simulink model "ABLF_SOC_benchmark"  (R2021b)
settings: Solver=FixedStepAuto  StartTime=0.0  StopTime=100  FixedStep=0.0001  RelTol=1e-3
values from neighbouring files (symbols this model uses):
  a = 2    [ABLF_SLDO_benchmark_Start.m]    (also in ABLF_SOC_benchmark_Start.m)
  amp = pi/2    (= 1.57079632679)    [ABLF_SLDO_benchmark_Start.m]    (also in ABLF_SOC_benchmark_Start.m)
  f1 = 0    [ABLF_SLDO_benchmark_Start.m]    (also in ABLF_SOC_benchmark_Start.m)
  g1 = 1    [ABLF_SLDO_benchmark_Start.m]    (also in ABLF_SOC_benchmark_Start.m)
  g2 = Kt/J    (= 0.530555555556)    [ABLF_SLDO_benchmark_Start.m]    (also in ABLF_SOC_benchmark_Start.m)
  g3 = 1/L    (= 333.333333333)    [ABLF_SLDO_benchmark_Start.m]    (also in ABLF_SOC_benchmark_Start.m)
  J = 1.8*10^(-2)    (= 0.018)    [ABLF_SLDO_benchmark_Start.m]    (also in ABLF_SOC_benchmark_Start.m)
  k = 2    [ABLF_SLDO_benchmark_Start.m]    (also in ABLF_SOC_benchmark_Start.m)
  k1 = 6.2718    [ABLF_SLDO_benchmark_Start.m]    (also in ABLF_SOC_benchmark_Start.m = 10)
  k2 = 2.3993e+03    (= 2399.3)    [ABLF_SLDO_benchmark_Start.m]    (also in ABLF_SOC_benchmark_Start.m = 1)
  k3 = 31.9167    [ABLF_SLDO_benchmark_Start.m]    (also in ABLF_SOC_benchmark_Start.m = 10)
  ka1 = kcl1 - (-amp)    (= -0.429203673205)    [ABLF_SLDO_benchmark_Start.m]    (also in ABLF_SOC_benchmark_Start.m = kcl1 - (-amp))
  kb1 = kcl2 - (amp)    (= 0.429203673205)    [ABLF_SLDO_benchmark_Start.m]    (also in ABLF_SOC_benchmark_Start.m = kcl2 - (amp))
  Ke = 9.55*10^(-3)    (= 0.00955)    [ABLF_SLDO_benchmark_Start.m]    (also in ABLF_SOC_benchmark_Start.m)
  Kt = 9.55*10^(-3)    (= 0.00955)    [ABLF_SLDO_benchmark_Start.m]    (also in ABLF_SOC_benchmark_Start.m)
  L = 0.003    [ABLF_SLDO_benchmark_Start.m]    (also in ABLF_SOC_benchmark_Start.m = 1)
  maxKd = 100    [ABLF_SOC_benchmark_Start.m]
  maxKi = 1    [ABLF_SOC_benchmark_Start.m]
  maxKp = 100    [ABLF_SOC_benchmark_Start.m]
  minKd = 0.001    [ABLF_SOC_benchmark_Start.m]
  minKi = 0.01    [ABLF_SOC_benchmark_Start.m]
  minKp = 0.01    [ABLF_SOC_benchmark_Start.m]
  mu1 = 1.8    [ABLF_SLDO_benchmark_Start.m]    (also in ABLF_SOC_benchmark_Start.m)
  optimPeriod = 0.5    [ABLF_SOC_benchmark_Start.m]
  OVLim = 0.15    [ABLF_SOC_benchmark_Start.m]
  R = 0.21    [ABLF_SLDO_benchmark_Start.m]    (also in ABLF_SOC_benchmark_Start.m)
  refSignalPeriod = 0.5    [ABLF_SOC_benchmark_Start.m]
  resetThreshold = 0.1    [ABLF_SOC_benchmark_Start.m]
  t2 = 0.012    [ABLF_SLDO_benchmark_Start.m]    (also in ABLF_SOC_benchmark_Start.m = 0.0005)
  t3 = 0.012    [ABLF_SLDO_benchmark_Start.m]    (also in ABLF_SOC_benchmark_Start.m = 0.01)
  TSLim = 0.1    [ABLF_SOC_benchmark_Start.m]
  W1 = 0.1    [ABLF_SOC_benchmark_Start.m]
  W2 = 1    [ABLF_SOC_benchmark_Start.m]
  W3 = 0.109    [ABLF_SOC_benchmark_Start.m]
undefined symbols (not defined in the file or in its folder): DiscIntNeverNeededParam
libraries: dspmathops x2
settings Model: Creator=mcald  LastModifiedBy=mcald
settings DataIOCC: ReturnWorkspaceOutputs=off

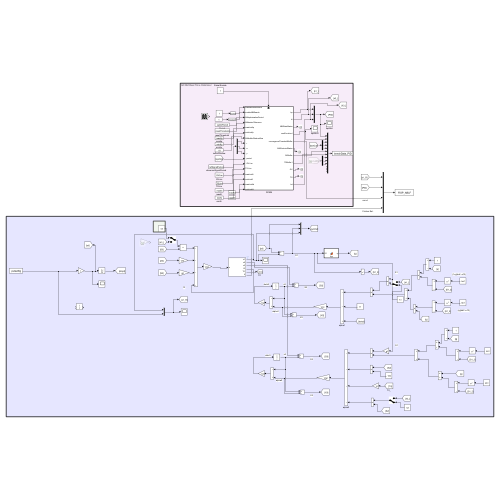
[thumbnail: Simulink's stored preview of the top-level diagram]
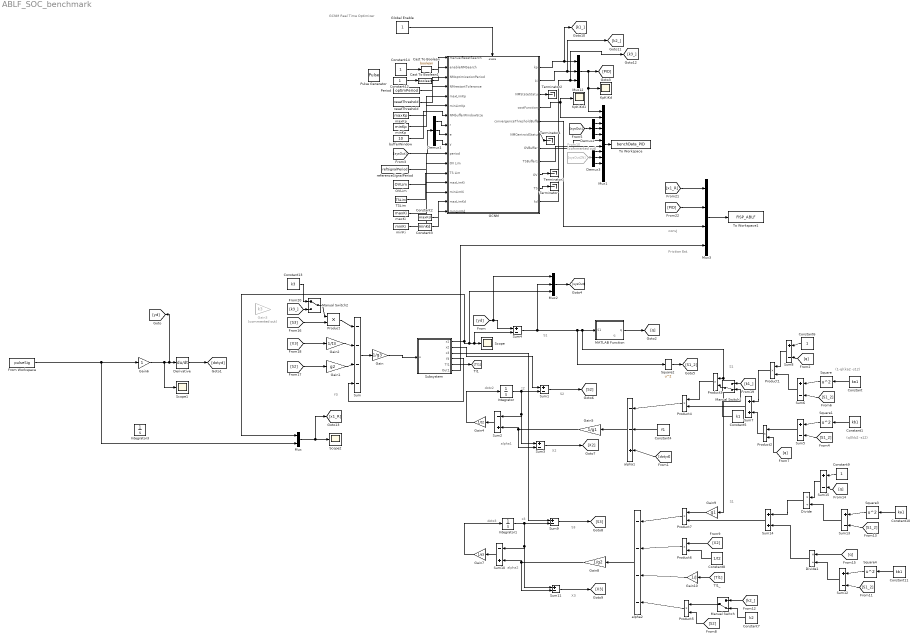
== system ABLF_SOC_benchmark ==
  note: Friction Est.
  note: convJ
  note: GCNM Real Time Optimizer
  note: S1
  note: alpha2
  note: S2
  note: z3
  note: f3
  note: dotz3
  note: (q)(kb2 -s12)
  note: X3
  note: S3
  note: S1
  note: S1
  note: q
  note: z2
  note: X2
  note: dotz2
  note: alpha1
  note: (1-q)(ka2 -s12)
  Cast To Boolean : DataTypeConversion  OutDataTypeStr=boolean
  Cast To Boolean1 : DataTypeConversion  OutDataTypeStr=boolean
  Constant : Constant  Value=ka1
  Constant1 : Constant  Value=kb1
  Constant10 : Constant  Value=ka1
  Constant11 : Constant  Value=kb1
  Constant12 : Constant  OutDataTypeStr=boolean
  Constant13 : Constant  Value=k3
  Constant14 : Constant
  Constant2 : Constant  Value=maxKd
  Constant3 : Constant  Value=minKd
  Constant4 : Constant  Value=f1
  Constant5 : Constant  Value=k1
  Constant6 : Constant
  Constant7 : Constant  Value=k2
  Constant8 : Constant  Value=1/t2
  Constant9 : Constant
  Demux1 : Demux  Outputs=3
  Demux2 : Demux  Outputs=3
  Demux3 : Demux  Outputs=3
  Derivative : Derivative
  Divide : Product  Inputs=*/
  Divide1 : Product  Inputs=*/
  From Workspace : FromWorkspace  VariableName=pulseSig
  From10 : From  Commented=on  GotoTag=sysOutZN
  GCNM : Subsystem
  Gain : Gain  Gain=1/g3
  Gain1 : Gain  Gain=g2
  Gain10 : Gain  Gain=1/J
  Gain2 : Gain  Gain=1/t3
  Gain3 : Gain  Commented=on  Gain=k3
  Gain4 : Gain  Gain=1/t2
  Gain5 : Gain  Gain=1/g1
  Gain6 : Gain
  Gain7 : Gain  Gain=1/t3
  Gain8 : Gain  Gain=1/g2
  Gain9 : Gain  Gain=g1
  Global Enable : Constant
  Integrator : Integrator  InitialCondition=-5.0078
  Integrator1 : Integrator  InitialCondition=-2094.2231
  Integrator3 : Integrator  InitialCondition=0.1
  KpKiKd : Scope
  KpKiKd1 : Scope
  MATLAB Function : MATLAB Function  TreatAsAtomicUnit=on
  Manual Switch : ManualSwitch  CurrentSetting=0
  Manual Switch1 : ManualSwitch  CurrentSetting=0
  Manual Switch2 : ManualSwitch
  Mux : Mux  Inputs=2
  Mux1 : Mux  Inputs=12
  Mux12 : Mux  Inputs=3
  Mux2 : Mux  Inputs=3
  Mux3 : Mux
  OVLim : Constant  Value=OVLim
  Period : Constant  Value=optimPeriod  OutDataTypeStr=double
  Product{,1..7} (8 alike) : Product
  Pulse Generator : DiscretePulseGenerator  PulseType=Time based  Period=20  PulseWidth=0.1
  Scope : Scope
  Scope1 : Scope
  Scope2 : Scope
  Square{,1..4} (5 alike) : Math  Operator=square  SaturateOnIntegerOverflow=on
  Subsystem : Subsystem
  Sum : Sum  Inputs=-|-|-|-
  Sum{1,3..6,8..9,11..13,15} (11 alike) : Sum  Inputs=+|-
  Sum10 : Sum  Inputs=-|+
  Sum14 : Sum  Inputs=+|+
  Sum2 : Sum  Inputs=-|+
  Sum7 : Sum  Inputs=+|+
  TSLim : Constant  Value=TSLim
  Terminator{,1..2,4} (4 alike) : Terminator
  To Workspace : ToWorkspace  VariableName=benchData_PID  SaveFormat=Timeseries  SampleTime=-1
  To Workspace1 : ToWorkspace  VariableName=FISP_ABLF  SaveFormat=Timeseries  SampleTime=-1
  alpha1 : Sum  Inputs=-|-|+
  alpha2 : Sum  Inputs=-|-|-|-
  bufferWindow : Constant  Value=10  OutDataTypeStr=uint16
  maxKi : Constant  Value=maxKi  VectorParams1D=off  OutDataTypeStr=double
  maxKp : Constant  Value=maxKp  OutDataTypeStr=double
  minKi : Constant  Value=minKi  OutDataTypeStr=double
  minKp : Constant  Value=minKp  OutDataTypeStr=double
  referenceSignalPeriod : Constant  Value=refSignalPeriod
  resetThreshold : Constant  Value=resetThreshold
  wires:
  GCNM/9(OV) -> Terminator1/1
  Constant2/1 -> GCNM/16(maxLimKd)
  maxKp/1 -> GCNM/5(maxLimKp)
  Demux3/3 -> Mux1/10
  GCNM/3(NMStateStatus) -> Terminator2/1
  minKp/1 -> GCNM/6(minLimKp)
  Constant3/1 -> GCNM/17(minLimKd)
  [sysOut] -> Demux1/1
  bufferWindow/1 -> GCNM/7(NMbufferWindowSize)
  GCNM/6(NMCentroidStatus) -> Terminator4/1
  Cast To Boolean1/1 -> GCNM/2(enableNMSearch)
  Mux1/1 -> To Workspace/1
  OVLim/1 -> GCNM/12("  OV Lim")
  Demux3/2 -> Mux1/9
  Constant12/1 -> Cast To Boolean1/1
  From10/1 -> Demux3/1
  GCNM/4(costFunctionJ) -> Mux1/2, KpKiKd1/1
  Demux3/1 -> Mux1/8
  GCNM/7(OVBuffer) -> Mux1/6
  GCNM/8(TSBuffer1) -> Mux1/7
  GCNM/11(kd) -> [k3_], Mux12/3
  Demux2/3 -> Mux1/5
  TSLim/1 -> GCNM/13(TS Lim)
  GCNM/1("  kp") -> [k1_], Mux12/1
  referenceSignalPeriod/1 -> GCNM/11("  period")
  Mux12/1 -> Mux1/1, KpKiKd/1, [PID]
  Demux1/3 -> GCNM/10("  y")
  GCNM/10(TS) -> Terminator/1
  Cast To Boolean/1 -> GCNM/1(manualResetSearch)
  Demux2/1 -> Mux1/3
  Demux1/1 -> GCNM/8("  r")
  resetThreshold/1 -> GCNM/4(NMrestartTolerance)
  Demux2/2 -> Mux1/4
  maxKi/1 -> GCNM/14(maxLimKi)
  Global Enable/1 -> GCNM/Enable
  Demux1/2 -> GCNM/9("  e")
  Period/1 -> GCNM/3(NMoptimizationPeriod)
  GCNM/2("  ki") -> [k2_], Mux12/2
  minKi/1 -> GCNM/15(minLimKi)
  Constant14/1 -> Cast To Boolean/1
  [sysOut] -> Demux2/1
  [q] -> Sum8/2
  Sum7/1 -> Product4/2
  Constant1/1 -> Square1/1
  MATLAB Function/1(q) -> [q]
  [S1_2] -> Sum12/2
  Subsystem/4(f3) -> Sum/4
  Gain5/1 -> Sum2/2, Sum3/2
  [Tl1] -> Gain10/1
  Constant/1 -> Square/1
  [S2] -> Gain1/1
  Divide/1 -> Sum14/1
  Square3/1 -> Sum13/1
  Square2/1 -> [S1_2]
  [q] -> Divide1/1
  [X3] -> Gain2/1
  Constant11/1 -> Square4/1
  Subsystem/3(x3) -> Sum9/1
  Mux/1 -> [x1_R], Scope2/1
  Sum1/1 -> [S2]
  [q] -> Sum15/2
  Gain9/1 -> Product7/1
  [X2] -> Product6/1
  Sum11/1 -> [X3]
  Constant8/1 -> Product6/2
  Subsystem/2(x2) -> Sum1/1
  [yd] -> Mux2/1, Sum4/1
  Sum15/1 -> Divide/1
  [S1_2] -> Sum13/2
  Constant9/1 -> Sum15/1
  Constant6/1 -> Sum8/1
  Divide1/1 -> Sum14/2
  Product7/1 -> alpha2/1
  Product5/1 -> alpha2/4
  [S2] -> Product5/2
  Gain8/1 -> Sum10/2, Sum11/2
  Square1/1 -> Sum5/1
  Gain7/1 -> Integrator1/1
  Integrator1/1 -> Sum11/1, Sum10/1, Sum9/2
  Product2/1 -> Sum7/2
  Product1/1 -> Sum7/1
  Product6/1 -> alpha2/2
  alpha1/1 -> Gain5/1
  alpha2/1 -> Gain8/1
  Sum10/1 -> Gain7/1
  Sum5/1 -> Product2/1
  Integrator/1 -> Sum3/1, Sum2/1, Sum1/2
  Sum9/1 -> [S3]
  Subsystem/5(Tl1) -> [Tl1]
  [S1_2] -> Sum6/2
  [q] -> Product2/2
  Product4/1 -> alpha1/1
  Sum4/1 -> Square2/1, Gain9/1, Product3/1, MATLAB Function/1(S1), Mux2/2
  Sum3/1 -> [X2]
  Gain2/1 -> Sum/2
  Gain6/1 -> Derivative/1, [yd], Scope1/1
  Derivative/1 -> [dotyd]
  [S1_2] -> Sum5/2
  Square4/1 -> Sum12/1
  Constant4/1 -> alpha1/2
  Gain/1 -> Subsystem/1(u)
  Sum6/1 -> Product1/2
  Sum8/1 -> Product1/1
  Sum12/1 -> Divide1/2
  From Workspace/1 -> Mux/2, Gain6/1
  Gain1/1 -> Sum/3
  Gain4/1 -> Integrator/1
  Product/1 -> Sum/1
  Sum/1 -> Gain/1
  Mux2/1 -> [sysOut]
  Sum2/1 -> Gain4/1
  [dotyd] -> alpha1/3
  Square/1 -> Sum6/1
  Sum13/1 -> Divide/2
  Sum14/1 -> Product7/2
  Product3/1 -> Product4/1
  [S3] -> Product/2
  Constant10/1 -> Square3/1
  Gain10/1 -> alpha2/3
  Subsystem/1(x1) -> Mux2/3, Sum4/2, Scope/1, Mux/1
  Mux3/1 -> To Workspace1/1
  [x1_R] -> Mux3/1
  [PID] -> Mux3/2
  GCNM/5(convergenceThresholdBuffer) -> Mux3/3
  Subsystem/6(Out1) -> Mux3/4
  Manual Switch/1 -> Product5/1
  [k2_] -> Manual Switch/1
  Constant7/1 -> Manual Switch/2
  Manual Switch1/1 -> Product3/2
  [k1_] -> Manual Switch1/1
  Constant5/1 -> Manual Switch1/2
  [k3_] -> Manual Switch2/2
  Constant13/1 -> Manual Switch2/1
  Manual Switch2/1 -> Product/1

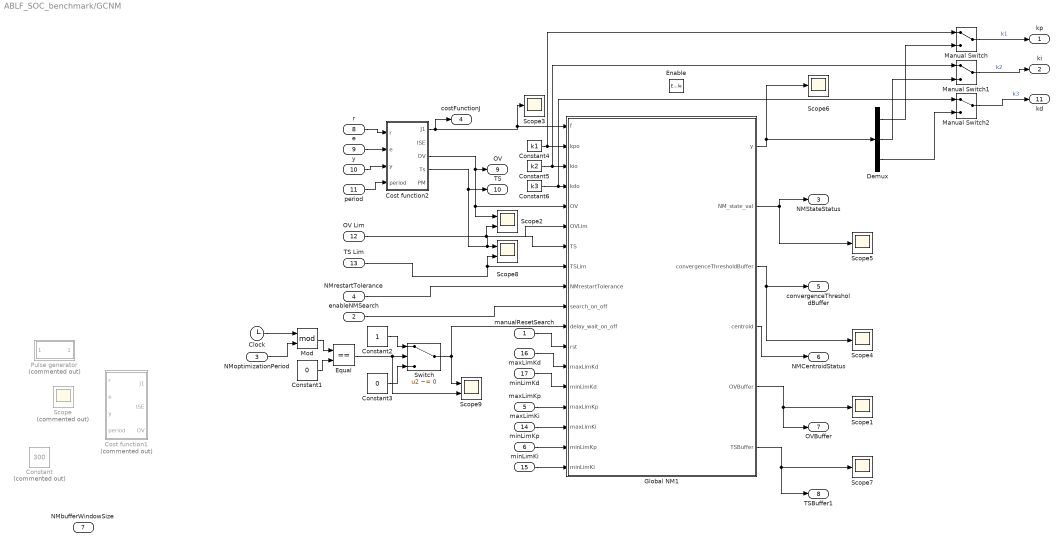
== system ABLF_SOC_benchmark/GCNM ==
  manualResetSearch : Inport  OutDataTypeStr=boolean
  enableNMSearch : Inport  Port=2  OutDataTypeStr=boolean
  NMoptimizationPeriod : Inport  Port=3  OutDataTypeStr=double
  NMrestartTolerance : Inport  Port=4
  maxLimKp : Inport  Port=5  OutDataTypeStr=double
  minLimKp : Inport  Port=6  OutDataTypeStr=double
  NMbufferWindowSize : Inport  Port=7  OutDataTypeStr=uint16
  "  r" : Inport  Port=8  OutDataTypeStr=double
  "  e" : Inport  Port=9  OutDataTypeStr=double
  "  y" : Inport  Port=10  OutDataTypeStr=double
  "  period" : Inport  Port=11  OutDataTypeStr=double
  "  OV Lim" : Inport  Port=12  OutDataTypeStr=double
  TS Lim : Inport  Port=13  OutDataTypeStr=double
  maxLimKi : Inport  Port=14  OutDataTypeStr=double
  minLimKi : Inport  Port=15  OutDataTypeStr=double
  maxLimKd : Inport  Port=16
  minLimKd : Inport  Port=17
  Enable : EnablePort
  Clock : Clock
  Constant : Constant  Commented=on  Value=300
  Constant1 : Constant  Value=0
  Constant2 : Constant
  Constant3 : Constant  Value=0
  Constant4 : Constant  Value=k1
  Constant5 : Constant  Value=k2
  Constant6 : Constant  Value=k3
  Cost function1 : Subsystem  Commented=on
  Cost function2 : Subsystem
  Demux : Demux  Outputs=3
  Equal : RelationalOperator  Operator===  RndMeth=Simplest
  Global NM1 : MATLAB Function  TreatAsAtomicUnit=on
  Manual Switch : ManualSwitch
  Manual Switch1 : ManualSwitch
  Manual Switch2 : ManualSwitch
  Mod : Math  Operator=mod  SaturateOnIntegerOverflow=on
  Pulse generator : Subsystem  Commented=on
  Scope : Scope  Commented=on
  Scope{1,3..7} (6 alike) : Scope
  Scope2 : Scope  NumInputPorts=2
  Scope8 : Scope  NumInputPorts=2
  Scope9 : Scope  NumInputPorts=2
  Switch : Switch  Criteria=u2 ~= 0
  "  kp" : Outport  OutDataTypeStr=double
  "  ki" : Outport  Port=2  OutDataTypeStr=double
  NMStateStatus : Outport  Port=3  OutDataTypeStr=double
  costFunctionJ : Outport  Port=4  OutDataTypeStr=double
  convergenceThresholdBuffer : Outport  Port=5  OutDataTypeStr=double
  NMCentroidStatus : Outport  Port=6  OutDataTypeStr=double
  OVBuffer : Outport  Port=7  OutDataTypeStr=double
  TSBuffer1 : Outport  Port=8  OutDataTypeStr=double
  OV : Outport  Port=9  OutDataTypeStr=double
  TS : Outport  Port=10  OutDataTypeStr=double
  kd : Outport  Port=11
  wires:
  NMrestartTolerance/1 -> Global NM1/9(NMrestartTolerance)
  manualResetSearch/1 -> Global NM1/12(rst)
  enableNMSearch/1 -> Global NM1/10(search_on_off)
  minLimKp/1 -> Global NM1/17(minLimKp)
  maxLimKp/1 -> Global NM1/15(maxLimKp)
  Global NM1/2(NM_state_val) -> NMStateStatus/1, Scope5/1
  Global NM1/3(convergenceThresholdBuffer) -> convergenceThresholdBuffer/1, Scope4/1
  Global NM1/4(centroid) -> NMCentroidStatus/1
  Global NM1/1(y) -> Scope6/1, Demux/1
  Constant5/1 -> Manual Switch1/1, Global NM1/3(kio)
  Cost function2/3(OV) -> OV/1, Scope2/1, Global NM1/5(OV)
  "  y"/1 -> Cost function2/3(y)
  "  e"/1 -> Cost function2/2(e)
  "  r"/1 -> Cost function2/1(r)
  Global NM1/5(OVBuffer) -> OVBuffer/1, Scope1/1
  "  period"/1 -> Cost function2/4(period)
  "  OV Lim"/1 -> Scope2/2, Global NM1/6(OVLim)
  Cost function2/4(Ts) -> TS/1, Global NM1/7(TS), Scope8/1
  TS Lim/1 -> Scope8/2, Global NM1/8(TSLim)
  Global NM1/6(TSBuffer) -> TSBuffer1/1, Scope7/1
  Cost function2/1(J1) -> Scope3/1, Global NM1/1(f), costFunctionJ/1
  Clock/1 -> Mod/1
  NMoptimizationPeriod/1 -> Mod/2
  Constant1/1 -> Equal/2
  Mod/1 -> Equal/1
  Constant2/1 -> Switch/1
  Constant3/1 -> Switch/3
  Switch/1 -> Scope9/1, Global NM1/11(delay_wait_on_off)
  Equal/1 -> Scope9/2, Switch/2
  maxLimKi/1 -> Global NM1/16(maxLimKi)
  minLimKi/1 -> Global NM1/18(minLimKi)
  maxLimKd/1 -> Global NM1/13(maxLimKd)
  minLimKd/1 -> Global NM1/14(minLimKd)
  Constant6/1 -> Manual Switch2/1, Global NM1/4(kdo)
  Constant4/1 -> Manual Switch/1, Global NM1/2(kpo)
  Manual Switch/1 -> "  kp"/1  "k1"
  Manual Switch2/1 -> kd/1  "k3"
  Manual Switch1/1 -> "  ki"/1  "k2"
  Demux/1 -> Manual Switch/2
  Demux/2 -> Manual Switch1/2
  Demux/3 -> Manual Switch2/2

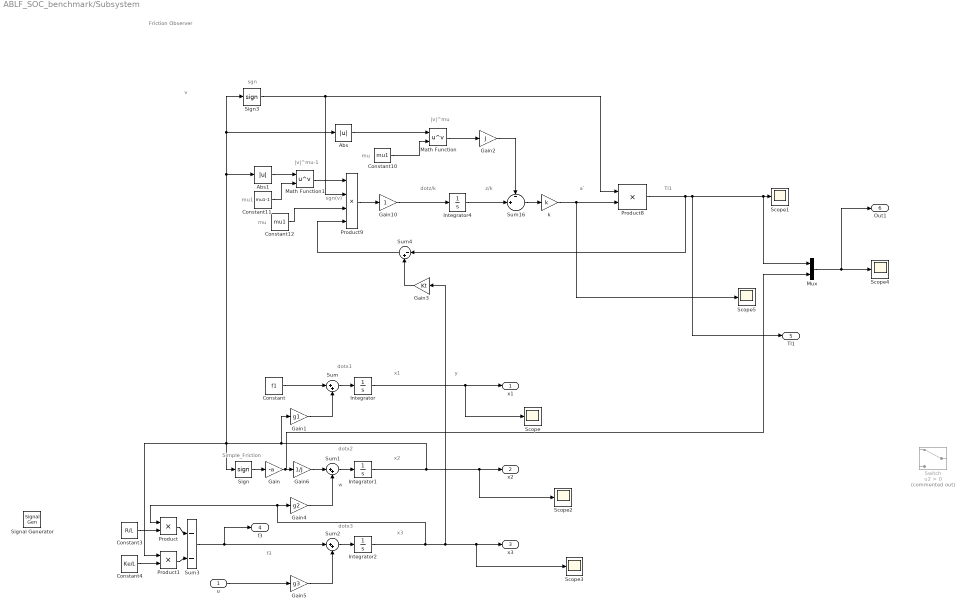
== system ABLF_SOC_benchmark/Subsystem ==
  note: Simple_Friction
  note: w
  note: f3
  note: y
  note: x1
  note: dotx1
  note: dotx2
  note: x2
  note: dotx3
  note: x3
  note: mu1
  note: dotz/k
  note: v
  note: mu
  note: a`
  note: z/k
  note: sgn
  note: Friction Observer
  note: mu
  note: |v|^mu-1
  note: sgn(v)
  note: |v|^mu
  note: Tl1
  u : Inport
  Abs : Abs
  Abs1 : Abs
  Constant : Constant  Value=f1
  Constant10 : Constant  Value=mu1
  Constant11 : Constant  Value=mu1-1
  Constant12 : Constant  Value=mu1
  Constant3 : Constant  Value=R/L
  Constant4 : Constant  Value=Ke/L
  Gain : Gain  Gain=-a
  Gain1 : Gain  Gain=g1
  Gain10 : Gain
  Gain2 : Gain  Gain=J
  Gain3 : Gain  Gain=Kt
  Gain4 : Gain  Gain=g2
  Gain5 : Gain  Gain=g3
  Gain6 : Gain  Gain=1/J
  Integrator : Integrator  InitialCondition=0.1
  Integrator1 : Integrator  InitialCondition=0.1
  Integrator2 : Integrator  InitialCondition=0.1
  Integrator4 : Integrator  InitialCondition=1
  Math Function : Math  Operator=pow  SaturateOnIntegerOverflow=on
  Math Function1 : Math  Operator=pow  SaturateOnIntegerOverflow=on
  Mux : Mux  Inputs=2
  Product : Product
  Product1 : Product
  Product8 : Product
  Product9 : Product  Inputs=4
  Scope{,1..5} (6 alike) : Scope
  Sign : Signum
  Sign3 : Signum
  Signal Generator : SignalGenerator  WaveForm=square  Amplitude=pi/2  Frequency=0.1  Units=rad/sec
  Sum : Sum  Inputs=|++
  Sum1 : Sum  Inputs=|++
  Sum16 : Sum  Inputs=-|+||
  Sum2 : Sum  Inputs=|++
  Sum3 : Sum  Inputs=-|-
  Sum4 : Sum  Inputs=|-+
  Switch : Switch  Commented=on  Criteria=u2 > Threshold
  k : Gain  Gain=k
  x1 : Outport
  x2 : Outport  Port=2
  x3 : Outport  Port=3
  f3 : Outport  Port=4
  Tl1 : Outport  Port=5
  Out1 : Outport  Port=6
  wires:
  Gain1/1 -> Sum/2
  Gain5/1 -> Sum2/2
  Integrator/1 -> Scope/1, x1/1
  Sum2/1 -> Integrator2/1
  Sum3/1 -> f3/1, Sum2/1
  Constant/1 -> Sum/1
  Sum1/1 -> Integrator1/1
  Integrator2/1 -> Gain3/1, Scope3/1, x3/1, Product/1, Gain4/1
  Sum/1 -> Integrator/1
  Constant3/1 -> Product/2
  Product/1 -> Sum3/1
  Product1/1 -> Sum3/2
  Constant4/1 -> Product1/2
  Integrator4/1 -> Sum16/2
  Abs1/1 -> Math Function1/1
  Math Function1/1 -> Product9/1
  Abs/1 -> Math Function/1
  Product9/1 -> Gain10/1
  Sum16/1 -> k/1
  Gain10/1 -> Integrator4/1
  Sign3/1 -> Product9/2, Product8/1
  Constant12/1 -> Product9/3
  Constant10/1 -> Math Function/2
  k/1 -> Scope5/1, Product8/2
  Constant11/1 -> Math Function1/2
  Sign/1 -> Gain/1
  Gain4/1 -> Sum1/2
  u/1 -> Gain5/1
  Math Function/1 -> Gain2/1
  Gain2/1 -> Sum16/1
  Mux/1 -> Out1/1, Scope4/1
  Product8/1 -> Sum4/1, Tl1/1, Mux/1, Scope1/1
  Integrator1/1 -> Gain1/1, Abs1/1, Abs/1, Sign3/1, Sign/1, Product1/1, Scope2/1, x2/1
  Gain3/1 -> Sum4/2
  Sum4/1 -> Product9/4
  Gain6/1 -> Sum1/1
  Gain/1 -> Mux/2, Gain6/1

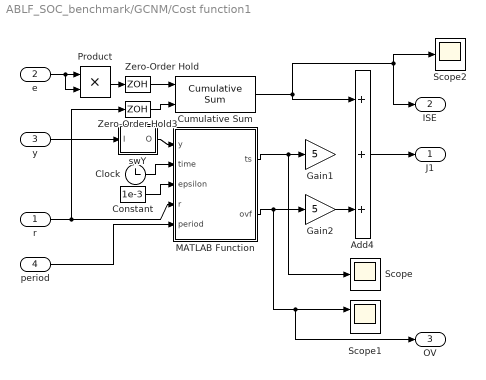
== system ABLF_SOC_benchmark/GCNM/Cost function1 ==
  r : Inport
  e : Inport  Port=2
  y : Inport  Port=3
  period : Inport  Port=4
  Add4 : Sum  Inputs=+++
  Clock : Clock
  Constant : Constant  Value=1e-3
  Cumulative Sum : dspmathops/Cumulative Sum  dim=Channels (running sum)  InputProcessing=Columns as channels (frame based)  reset_popup=Falling edge  roundingMode=Floor  overflowMode=off  outputDataTypeStr=Inherit: Same as accumulator  outputMin=[]  outputMax=[]  outputLastDataTypeStr=Inherit: Same as accumulator
  Gain1 : Gain  Gain=5
  Gain2 : Gain  Gain=5
  MATLAB Function : MATLAB Function  TreatAsAtomicUnit=on
  Product : Product
  Scope : Scope
  Scope1 : Scope  NumInputPorts=2
  Scope2 : Scope
  Zero-Order Hold : ZeroOrderHold  SampleTime=-1
  Zero-Order Hold3 : ZeroOrderHold  SampleTime=-1
  swY : Subsystem
  J1 : Outport
  ISE : Outport  Port=2
  OV : Outport  Port=3
  wires:
  period/1 -> MATLAB Function/5(period)
  Gain2/1 -> Add4/3
  Add4/1 -> J1/1
  y/1 -> swY/1(I)
  Constant/1 -> MATLAB Function/3(epsilon)
  Product/1 -> Zero-Order Hold/1
  Clock/1 -> MATLAB Function/2(time)
  swY/1(O) -> MATLAB Function/1(y)
  MATLAB Function/2(ovf) -> Gain2/1, Scope1/1, OV/1
  r/1 -> MATLAB Function/4(r), Zero-Order Hold3/1
  Zero-Order Hold/1 -> Cumulative Sum/1
  MATLAB Function/1(ts) -> Gain1/1, Scope/1
  e/1 -> Product/1, Product/2
  Zero-Order Hold3/1 -> Cumulative Sum/2
  Cumulative Sum/1 -> Scope2/1, ISE/1, Add4/1

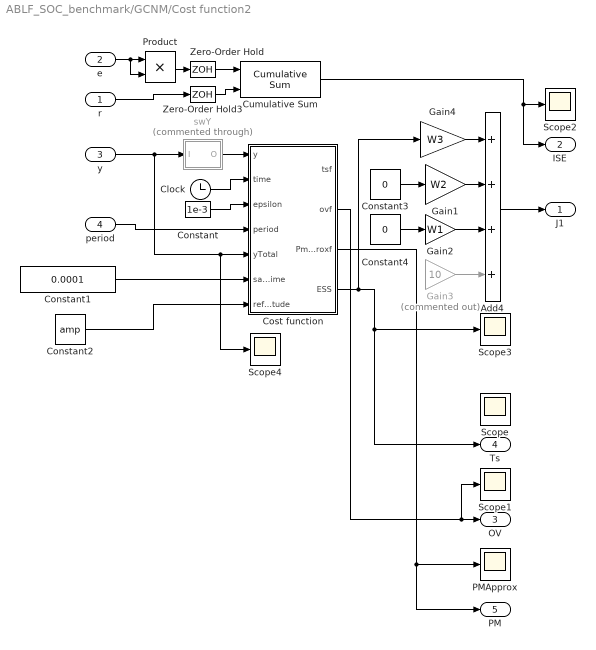
== system ABLF_SOC_benchmark/GCNM/Cost function2 ==
  r : Inport
  e : Inport  Port=2
  y : Inport  Port=3
  period : Inport  Port=4
  Add4 : Sum  Inputs=++++
  Clock : Clock
  Constant : Constant  Value=1e-3
  Constant1 : Constant  Value=0.0001
  Constant2 : Constant  Value=amp
  Constant3 : Constant  Value=0
  Constant4 : Constant  Value=0
  Cost function : MATLAB Function  TreatAsAtomicUnit=on
  Cumulative Sum : dspmathops/Cumulative Sum  dim=Channels (running sum)  InputProcessing=Columns as channels (frame based)  reset_popup=Falling edge  roundingMode=Floor  overflowMode=off  outputDataTypeStr=Inherit: Same as accumulator  outputMin=[]  outputMax=[]  outputLastDataTypeStr=Inherit: Same as accumulator
  Gain1 : Gain  Gain=W2
  Gain2 : Gain  Gain=W1
  Gain3 : Gain  Commented=on  Gain=10
  Gain4 : Gain  Gain=W3
  PMApprox : Scope
  Product : Product
  Scope{,1..4} (5 alike) : Scope
  Zero-Order Hold : ZeroOrderHold  SampleTime=-1
  Zero-Order Hold3 : ZeroOrderHold  SampleTime=-1
  swY : Subsystem  Commented=through
  J1 : Outport
  ISE : Outport  Port=2
  OV : Outport  Port=3
  Ts : Outport  Port=4
  PM : Outport  Port=5
  wires:
  Cumulative Sum/1 -> ISE/1, Scope2/1
  Zero-Order Hold3/1 -> Cumulative Sum/2
  e/1 -> Product/2, Product/1
  Zero-Order Hold/1 -> Cumulative Sum/1
  r/1 -> Zero-Order Hold3/1
  swY/1(O) -> Cost function/1(y)
  Clock/1 -> Cost function/2(time)
  Product/1 -> Zero-Order Hold/1
  Constant/1 -> Cost function/3(epsilon)
  y/1 -> Scope4/1, Cost function/5(yTotal), swY/1(I)
  Add4/1 -> J1/1
  Gain2/1 -> Add4/3
  period/1 -> Cost function/4(period)
  Constant1/1 -> Cost function/6(samplingTime)
  Gain1/1 -> Add4/2
  Constant2/1 -> Cost function/7(refAmplitude)
  Gain3/1 -> Add4/4
  Cost function/2(ovf) -> Scope1/1, OV/1
  Cost function/3(PmAproxf) -> PM/1, PMApprox/1
  Gain4/1 -> Add4/1
  Cost function/4(ESS) -> Gain4/1, Ts/1, Scope3/1
  Constant3/1 -> Gain1/1
  Constant4/1 -> Gain2/1

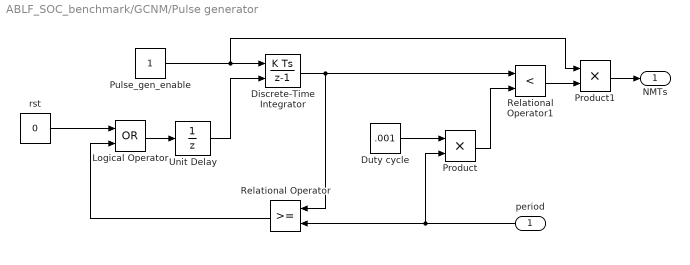
== system ABLF_SOC_benchmark/GCNM/Pulse generator ==
  period : Inport
  Discrete-Time Integrator : DiscreteIntegrator  ExternalReset=rising  SampleTime=-1  ICPrevOutput=DiscIntNeverNeededParam  ICPrevScaledInput=DiscIntNeverNeededParam
  Duty cycle : Constant  Value=.001
  Logical Operator : Logic  Operator=OR  AllPortsSameDT=off  OutDataTypeStr=boolean
  Product : Product  RndMeth=Zero
  Product1 : Product  RndMeth=Zero
  Pulse_gen_enable : Constant
  Relational Operator : RelationalOperator  OutDataTypeStr=boolean  RndMeth=Nearest
  Relational Operator1 : RelationalOperator  Operator=<  OutDataTypeStr=boolean  RndMeth=Nearest
  Unit Delay : UnitDelay  SampleTime=-1
  rst : Constant  Value=0
  NMTs : Outport
  wires:
  Pulse_gen_enable/1 -> Discrete-Time Integrator/1, Product1/1
  Unit Delay/1 -> Discrete-Time Integrator/2
  Duty cycle/1 -> Product/1
  Product/1 -> Relational Operator1/2
  Discrete-Time Integrator/1 -> Relational Operator/1, Relational Operator1/1
  period/1 -> Relational Operator/2, Product/2
  Logical Operator/1 -> Unit Delay/1
  rst/1 -> Logical Operator/1
  Relational Operator/1 -> Logical Operator/2
  Relational Operator1/1 -> Product1/2
  Product1/1 -> NMTs/1

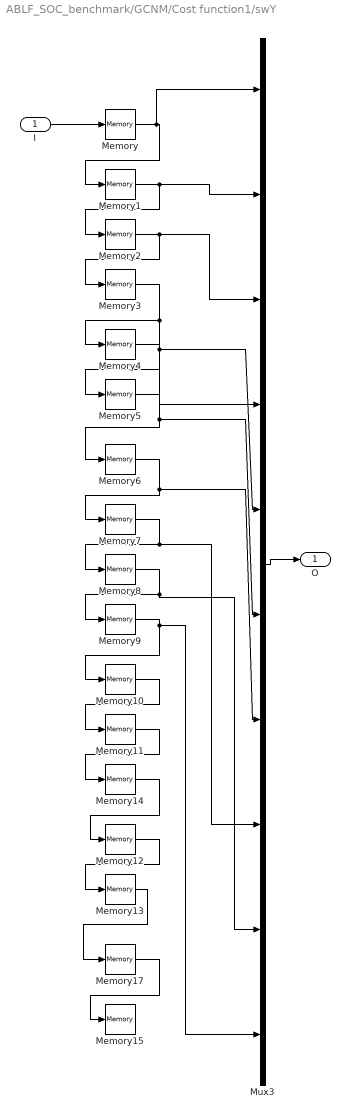
== system ABLF_SOC_benchmark/GCNM/Cost function1/swY ==
  I : Inport
  Memory{,1..15,17} (17 alike) : Memory
  Mux3 : Mux  Inputs=10
  O : Outport
  wires:
  Memory17/1 -> Memory15/1
  Memory7/1 -> Mux3/8, Memory8/1
  Memory/1 -> Mux3/1, Memory1/1
  Memory8/1 -> Mux3/9, Memory9/1
  I/1 -> Memory/1
  Memory2/1 -> Mux3/3, Memory3/1
  Memory10/1 -> Memory11/1
  Memory1/1 -> Mux3/2, Memory2/1
  Memory6/1 -> Mux3/7, Memory7/1
  Memory3/1 -> Mux3/4, Memory4/1
  Memory9/1 -> Mux3/10, Memory10/1
  Mux3/1 -> O/1
  Memory4/1 -> Mux3/5, Memory5/1
  Memory5/1 -> Mux3/6, Memory6/1
  Memory13/1 -> Memory17/1
  Memory12/1 -> Memory13/1
  Memory14/1 -> Memory12/1
  Memory11/1 -> Memory14/1

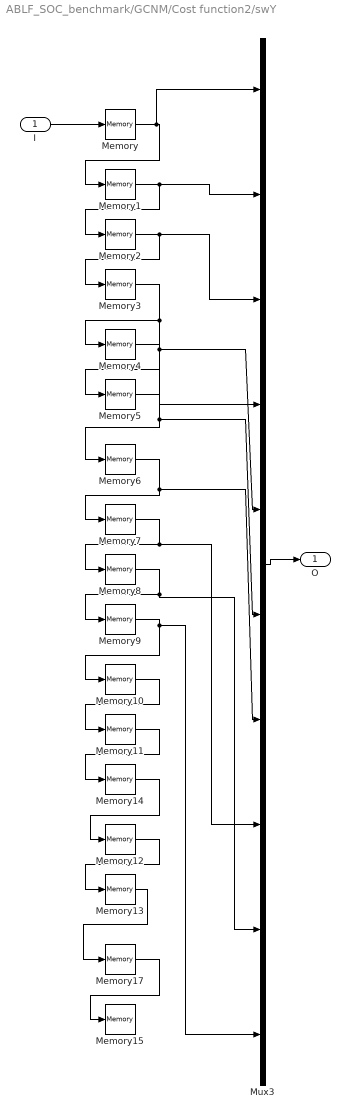
== system ABLF_SOC_benchmark/GCNM/Cost function2/swY ==
  I : Inport
  Memory{,1..15,17} (17 alike) : Memory
  Mux3 : Mux  Inputs=10
  O : Outport
  wires:
  Memory11/1 -> Memory14/1
  Memory14/1 -> Memory12/1
  Memory12/1 -> Memory13/1
  Memory13/1 -> Memory17/1
  Memory5/1 -> Memory6/1, Mux3/6
  Memory4/1 -> Memory5/1, Mux3/5
  Mux3/1 -> O/1
  Memory9/1 -> Memory10/1, Mux3/10
  Memory3/1 -> Memory4/1, Mux3/4
  Memory6/1 -> Memory7/1, Mux3/7
  Memory1/1 -> Memory2/1, Mux3/2
  Memory10/1 -> Memory11/1
  Memory2/1 -> Memory3/1, Mux3/3
  I/1 -> Memory/1
  Memory8/1 -> Memory9/1, Mux3/9
  Memory/1 -> Memory1/1, Mux3/1
  Memory7/1 -> Memory8/1, Mux3/8
  Memory17/1 -> Memory15/1

== matlab function ABLF_SOC_benchmark/GCNM/Cost function2/Cost function ==
  settings: updateMethod=DISCRETE
  data: y input; tsf output; time input; ovf output; epsilon input; period input; yTotal input; samplingTime input; refAmplitude input; PmAproxf output; ESS output
function [tsf,ovf,PmAproxf,ESS] = performance(y,time,epsilon,period,yTotal,samplingTime,refAmplitude)
        persistent OV tsFlag yHist counter ts PmAprox OV_1 ESS_1;
        
        %initialization state
          if isempty(OV)        
              OV=0;
              PmAprox=0;
              tsFlag=1;
              yHist=zeros(1,round(period/(2*samplingTime)));          
%               ts=0;
              counter=1;
              ts=0*samplingTime;
              tsf=0;
              OV_1=0;
              ESS=1;
              ESS_1=0;
          end
          
          yHist(counter)=yTotal;
          
          %overshoot and phase margin calculation 
%           OVCurrent=(max(y)-refAmplitude);
       
%           tsFlag=max(y);
%           if OVCurrent>OV
%               OV=OVCurrent;
%               ovf=OV;
%               OVPor=abs(OV)/refAmplitude+1e-3;     %overshoot percentage
% %               OVPor=abs(OV-refAmplitude+0.001)/refAmplitude;     %overshoot percentage
%               PmAprox= 100*( -log(OVPor)/ sqrt( pi^2+log(OVPor)^2 )); %approximated phase margin (based on second order system approximation)
%               PmAproxf=PmAprox;
%           else
%               ovf=OV;
%               PmAproxf=PmAprox;
%           end
          
          %calculate settling time each half of the period
          if mod(time,(period/2))==0    

    %       ESS=mean((abs(yHist( round((length(yHist)*8/10)):end)   )-refAmplitude));
            ESS=std((refAmplitude - abs(yHist( round((length(yHist)*9/10)):end)   )));
            ovf=abs((max((yHist))-(refAmplitude))/refAmplitude)+1e-3;
            ESS_1=ESS;
            OV_1=ovf;
            ts=converTimeInv(yHist,10,epsilon);
       %      yHist=zeros(1,round(period/2));
            
            tsf=ts*samplingTime;
            PmAproxf=0;
            counter=0;
          else
              ovf=OV_1;
              tsf=ts*samplingTime;
              PmAproxf=0;
              ESS=ESS_1;
          end
          
          
          if mod(time,period)==0    %restart constraints after each repetitive period
            ovf=OV_1;
            tsf=0;
            PmAproxf=0;
            ESS=0;
          else
              PmAproxf=0;
              ESS=ESS_1;
          end
          
          counter=counter+1;
          

end

== matlab function ABLF_SOC_benchmark/MATLAB Function ==
  data: S1 input; q output
function q = fcn(S1)
if S1 <= 0
    q = 0;
else  
    q = 1;
end

== matlab function ABLF_SOC_benchmark/GCNM/Global NM1 ==
  settings: updateMethod=DISCRETE
  data: f input; y output size=3; kpo input; kio input; kdo input; OV input; OVLim input; TS input; TSLim input; NM_state_val output; convergenceThresholdBuffer output; NMrestartTolerance input; centroid output; search_on_off input; delay_wait_on_off input; rst input; maxLimKd input; minLimKd input; OVBuffer output; maxLimKp input; maxLimKi input; minLimKp input; TSBuffer output; minLimKi input
%function [y, NM_state_val,convergenceThresholdBuffer,centroid,BiasRFState1ReflectionCoefficientBuffer]= fcn(f,kpo, kio,BiasRFState1ReflectionCoefficient,BiasRFState1ReflectionCoefficientLim,...
%                                                                                                            NMrestartTolerance, search_on_off, delay_wait_on_off, rst,maxLim,minLim)
function [y, NM_state_val,convergenceThresholdBuffer,centroid,OVBuffer,TSBuffer]= fcn(f,kpo, kio,kdo,OV,OVLim,TS,TSLim,...
                                                                                                           NMrestartTolerance, search_on_off, delay_wait_on_off, rst,maxLimKd,minLimKd,maxLimKp,maxLimKi,minLimKp,minLimKi)

% persistent count
persistent NM_state         %Integer definition for states, since enum is not supported
persistent Full_eval_count
persistent usual_delta      %5 percent deltas for non-zero terms
persistent zero_term_delta  %Even smaller delta for zero elements of x
persistent v fv v_r v_e v_m f_r v_c 
persistent yp               %last output when search was on
persistent delay_edge
persistent delay_wait_on_off_z
persistent f_old
persistent windowCounter convergenceThresholdStd gamma1Std gamma2Std delta1Std  ps1Std ps2Std delta2Std
persistent bufferJ bufferGamma1 bufferGamma2 bufferDelta1 bufferDelta2 bufferPS1 bufferPS2;

x=[kpo,kio,kdo];  %Initial conditions vector for kp and ki terms

%mead algorithm reset using normal distribution with 1000 choices of initial conditions for Nelder
n = 3;      %Input dimension - needs to be defined as a constant to keep Simulink port width inheretence happy
np1 = n+1;  %Simplex solid dimension
n_r = 1/n;  %Calculate reciprocal at compilation time for mean calculation

%Simplex update coefficients %Can be a function of dimension see Han2010
% alpha = 1;
% beta = 2;
% gamma = 0.5;
% delta = 0.5;

%Adaptive simplex search coefficients: Han2010
alpha = 1;%0.5;
beta = 1 + 2*n_r;%0.5 + 2*n_r;
gamma = 0.75 - 0.5*n_r;
delta = 1 - n_r;

bufferWindow=10;
%NM_state:  
    %0 - Initial   (Initialize vertices)
    %1 - FVE: Full vertex evaluation (with insertion sort after each evaluation)
    %2 - Insertion Sort (After Reflection, Expansion or Contraction Steps)
    %3 - Reflection Entry
    %4 - Reflection Evaluate
    %5 - Expansion
    %6 - Outside Contraction
    %7 - Inside Contraction
    %(8) - Shrink (Implicit on contraction outcome)

%Full_eval_count:
    %Number of initial vertices evaluated
    xin = x(:);         %Force xin to be a column vector
    coder.cinclude('<time.h>')   %% add the library time.c to the generated code
%initialization state of the Nelder Mead
    if isempty(NM_state)
        
        sd=0;
        sd=coder.ceval('time',[]);   %take the seed from the system current time
        rng(sd,'twister');           %initialize the seed of the system using current system seed

        delay_edge = 0;
        yp = xin;
        delay_wait_on_off_z = 0;
        convergenceThresholdStd=100;
        gamma1Std=1;
        gamma2Std=1;
        delta1Std=1;
        delta2Std=1;
        ps1Std=1;
        ps2Std=1;

        windowCounter=1; 
        bufferJ=zeros(1,bufferWindow);
        bufferGamma1=zeros(1,bufferWindow); 
        bufferGamma2=zeros(1,bufferWindow);
        bufferDelta1=zeros(1,bufferWindow); 
        bufferDelta2=zeros(1,bufferWindow); 
        bufferPS1=zeros(1,bufferWindow);
        bufferPS2=zeros(1,bufferWindow);
        
        v = zeros(n,np1);   %Initialize n+1 vertices for simplex
        fv = zeros(1,np1);  %function values at the vertices
        v_m = v(:,1);       %0 vector
        v_r = v_m;          %0 vector    
        v_e = v_m;          %0 vector
        v_c = v_m;          %0 vector
        f_r = 0;          %0 vector

%         usual_delta = 0.01; %original 0.07
        usual_delta = 0.1; %original 0.07
%         zero_term_delta = 0.000025;
        zero_term_delta = 0.0025;
        NM_state = 0;          %Initial state
        Full_eval_count = 1;   %No vertices evaulated, yet

        v(:,1) = xin;
        for j=1:n
            vt = xin;
            if vt(j) ~= 0
                vt(j) = (1 + usual_delta)*vt(j);
            else
                vt(j) = zero_term_delta;
            end
            v(:, j+1) = vt;
        end
        v(2,:)=v(2,:);
    end
    
    
% if (rst==1)  %%Reset the search (Forced reset by external source)
%         f_old = 0;
%         delay_edge = 0;
%         y = xin;
%         delay_wait_on_off_z = 0;
%         convergenceThresholdStd=0;
%        
%         windowCounter=1; 
%         bufferJ=zeros(1,bufferWindow);
%         bufferGamma1=zeros(1,bufferWindow); 
%         bufferGamma2=zeros(1,bufferWindow);
%         bufferDelta1=zeros(1,bufferWindow); 
%         bufferDelta2=zeros(1,bufferWindow); 
%         bufferPS1=zeros(1,bufferWindow);
%         bufferPS2=zeros(1,bufferWindow);
%         
%         v = zeros(n,np1);   %Initialize n+1 vertices for simplex
0%         fv = zeros(1,np1);  %function values at the vertices
%         v_m = v(:,1);       %0 vector
%         v_r = v_m;          %0 vector    
%         v_e = v_m;          %0 vector
%         v_c = v_m;          %0 vector
%         f_r = 0;          %0 vector
% 
%         usual_delta = 0.05;
%         zero_term_delta = 0.00025;
%         
% %         usual_delta = 0.1; %Use for force cross decoupling search
% %         zero_term_delta = 0.05; %Use for force cross decoupling search
% 
%         NM_state = 0;          %Initial state
%         Full_eval_count = 1;   %No vertices evaulated, yet
% 
%         v(:,1) = xin;
%         
%         for j=1:n
%             vt = xin;
%             if vt(j) ~= 0
%                 vt(j) = (1 + usual_delta)*vt(j);
%             else
%                 vt(j) = zero_term_delta;
%             end
%             v(:, j+1) = vt;
%         end
% end



%+++++++++++++ NM search enabling rising flank+++++++++++++++++++++++++++++
% if ((delay_wait_on_off_z == 1) && (delay_wait_on_off == 0))  %falling edge detection for delay_wait_on_off
if ((delay_wait_on_off_z == 0) && (delay_wait_on_off == 1)) %rising edge detection for delay_wait_on_off
    delay_edge = 1;    
    elseif ((delay_wait_on_off_z == 0) && (delay_wait_on_off == 0)) %while level is low
% elseif ((delay_wait_on_off_z == 1) && (delay_wait_on_off == 1)) %while level is high
    delay_edge = 0;
end
    
   
    
%%%++++++++++NM optimization algorithm execution if enable and rising flank are activated   
if ((search_on_off==1) && (delay_edge==1))  




    %restart initialization routine
    gammaCond=(gamma1Std>=OVLim );%|| gamma2Std>=BiasRFState2ReflectionCoefficientLim);
    deltaCond=(delta1Std>=TSLim);% || delta2Std>=ADVCIPowerSetpointState2Lim);
%     psCond=(ps1Std>=ADVCIPulseQualityDeviationState1Lim || ps2Std>=ADVCIPulseQualityDeviationState2Lim);
    if (abs(convergenceThresholdStd)<= NMrestartTolerance && (gammaCond==1) || deltaCond==1)% || psCond==1) )%&& v_m(1,:)~=0)   %fv(1)>-28       %redo void case, restart the search

           v = zeros(n,np1);   %Initialize n+1 vertices for simplex
           fv = zeros(1,np1);      %function values at the vertices
            v_m = v(:,1);       %0 vector
            v_r = v_m;          %0 vector    
            v_e = v_m;          %0 vector
            v_c = v_m;          %0 vector
            f_r = 0;            %0 vector

%             usual_delta = 0.005;
            usual_delta = 0.1;
            zero_term_delta = 0.025;
            NM_state = 0;          %Initial state
            Full_eval_count = 1;   %No vertices evaulated, yet

            %new initial condition for probabilistic restart
% %             v(:,1) = (maxLim*rand(2,1));
%             v(1,1) = (maxLimKp*rand(1,1));
%             v(2,1) = (maxLimKi*rand(1,1));
%             while ((v(1,1)>maxLim || v(1,1)<minLim) || (v(2,1)>maxLimKi || v(2,1)<minLimKi))==1
%                 v(:,1) = round(maxLim*rand(2,1))
%             end
%         v(:,1) = (maxLimKp*rand(2,1));
            v(1,1) = (maxLimKp*rand(1,1));
            v(2,1) = (maxLimKi*rand(1,1));
            v(3,1) = (maxLimKd*rand(1,1));
            while ((v(1,1)>maxLimKp || v(1,1)<minLimKp) || (v(2,1)>maxLimKi || v(2,1)<minLimKi) || (v(3,1)>maxLimKd || v(3,1)<minLimKd))==1
                v(1,1) = (maxLimKp*rand(1,1));
                v(2,1) = (maxLimKi*rand(1,1));
                v(3,1) = (maxLimKd*rand(1,1));
                v(:,1);
            end


            xin=v(:,1);

            for j=1:n
                vt = xin;
                if vt(j) ~= 0
                    vt(j) = (1 + usual_delta)*vt(j);
                else
                    vt(j) = zero_term_delta;
                end
                v(:, j+1) = vt;
            end   
        convergenceThresholdStd=1;


    end    


    %%%%%%%%%%%%%%%%%%%%%% Nelder Mead State selection  %%%%%%%%%%%%%%%%%%%%%%%     
        switch NM_state  
            case 0 %Vertices has just been initialized
              y = v(:, Full_eval_count); %Write out first vertex for evaluation
              NM_state = 1;

            case 1 %Full vertex evaluation  
                fv(Full_eval_count) = f; %costFunctionJ;  %Read evaluated function value

                j = Full_eval_count;  %New value came in, insert it into sorted list
                while ( (j>1) && (fv(j-1)>fv(j)) ) %Sort ascending
                   temp = fv(j-1);
                   fv(j-1) = fv(j);
                   fv(j) = temp;
                   temp = v(:, j-1);
                   v(:, j-1) = v(:, j); %Also sort corresponding (evaluated) vertices 
                   v(:, j) = temp;
                   j = j-1;
                end

                Full_eval_count = Full_eval_count + 1;            
                if (Full_eval_count <= (np1))
                    y = v(:, Full_eval_count);                
                else
                    Full_eval_count = Full_eval_count - 1; 
                    %NM_state = 3;   %Full vertex evaluation complete -> Reflection 
                    v_sum = xin*0;  %Initialize sum for mean calculation

                    for i=1:n
                        v_sum = v_sum + v(:, i);
                    end

                    v_m = v_sum*n_r; %Centroid
                    v_r  = v_m*(1+alpha) - alpha*v(:, end);
                    y  = v_r;
                    NM_state = 4;   %Reflection Evaluate
                end

            case 2 %Insertion Sort                        
                    j = Full_eval_count;  %New value came in, insert it into list
                       while ( (j>1) && (fv(j-1)>fv(j)) ) %Sort ascending
                           temp = fv(j-1);
                           fv(j-1) = fv(j);
                           fv(j) = temp;
                           temp = v(:, j-1);
                           v(:, j-1) = v(:, j); %Also sort corresponding (evaluated) vertices 
                           v(:, j) = temp;
                           j = j-1;
                       end
                       y  = v_r;
                    NM_state = 3;   %Reflection 

            case 3 %Reflection Entry
                    v_sum = xin*0;  %Initialize sum for mean calculation

                    for i=1:n
                        v_sum = v_sum + v(:, i);
                    end

                    v_m = v_sum*n_r; %Centroid
                    v_r  = v_m*(1+alpha) - alpha*v(:, np1);
                    y  = v_r;
                    NM_state = 4;   %Reflection Evaluate

            case 4 %Reflection Evaluate
                f_r = f; %costFunctionJ;
                if ( (f_r>fv(:, 1)) && (f_r<fv(:, n)) )
                    v(:, np1) = v_r;
                    fv(np1) = f_r;
                    %NM_state = 2;
                    j = Full_eval_count;  %New value came in, insert it into list
                    while ( (j>1) && (fv(j-1)>fv(j)) ) %Sort ascending
                       temp = fv(j-1);
                       fv(j-1) = fv(j);
                       fv(j) = temp;
                       temp = v(:, j-1);
                       v(:, j-1) = v(:, j); %Also sort corresponding (evaluated) vertices 
                       v(:, j) = temp;
                       j = j-1;
                    end
                    %%NM_state = 3;   %Reflection 

                    v_sum = xin*0;  %Initialize sum for mean calculation

                    for i=1:n
                        v_sum = v_sum + v(:, i);
                    end

                    v_m = v_sum*n_r; %Centroid
                    v_r  = v_m*(1+alpha) - alpha*v(:, np1);
                    y  = v_r;
                    NM_state = 4;    %Reflection Evaluate
                elseif (f_r<fv(:, 1))
                    v_e  = v_m*(1-beta) + beta*v_r; 
                    y  = v_e;
                    NM_state = 5;    %Expansion
                else
                    if ( (f_r>=fv(n)) && (f_r<fv(np1)) ) 
                        v_c  = v_m*(1-gamma) + gamma*v_r; 
                        NM_state = 6; %Outside Contraction
                    elseif (f_r>=fv(np1))  
                        v_c  = v_m*(1+gamma) - gamma*v_r; 
                        NM_state = 7; %Inside Contraction
                    end
                    y = v_c;
                end

            case 5 %Expansion
                f_e = f; %costFunctionJ;
                if (f_e<f_r)
                    v(:, end) = v_e;
                    fv(end) = f_e;
                    %NM_state = 2;
                        j = Full_eval_count;  %New value came in, insert it into list
                       while ( (j>1) && (fv(j-1)>fv(j)) ) %Sort ascending
                           temp = fv(j-1);
                           fv(j-1) = fv(j);
                           fv(j) = temp;
                           temp = v(:, j-1);
                           v(:, j-1) = v(:, j); %Also sort corresponding (evaluated) vertices 
                           v(:, j) = temp;
                           j = j-1;
                       end
                    %%NM_state = 3;   %Reflection 

                    v_sum = xin*0;  %Initialize sum for mean calculation

                    for i=1:n
                        v_sum = v_sum + v(:, i);
                    end

                    v_m = v_sum*n_r; %Centroid
                    v_r  = v_m*(1+alpha) - alpha*v(:, np1);
                    y  = v_r;
                    NM_state = 4;   %Reflection Evaluate
                 else
                    v(:, np1) = v_r;
                    fv(np1) = f_r;
                    %NM_state = 2;
                    j = Full_eval_count;  %New value came in, insert it into list
                   while ( (j>1) && (fv(j-1)>fv(j)) ) %Sort ascending
                       temp = fv(j-1);
                       fv(j-1) = fv(j);
                       fv(j) = temp;
                       temp = v(:, j-1);
                       v(:, j-1) = v(:, j); %Also sort corresponding (evaluated) vertices 
                       v(:, j) = temp;
                       j = j-1;
                   end

                   %%NM_state = 3;   %Reflection 

                    v_sum = xin*0;  %Initialize sum for mean calculation

                    for i=1:n
                        v_sum = v_sum + v(:, i);
                    end

                    v_m = v_sum*n_r; %Centroid
                    v_r  = v_m*(1+alpha) - alpha*v(:, np1);
                    y  = v_r;
                    NM_state = 4;   %Reflection Evaluate
                end

           case 6 %Contraction
               f_c = f;%costFunctionJ;
               if (f_c<f_r)
                   v(:, np1) = v_c;
                   fv(np1) = f_c;
                   %NM_state = 2;
                   j = Full_eval_count;  %New value came in, insert it into list
                   while ( (j>1) && (fv(j-1)>fv(j)) ) %Sort ascending
                       temp = fv(j-1);
                       fv(j-1) = fv(j);
                       fv(j) = temp;
                       temp = v(:, j-1);
                       v(:, j-1) = v(:, j); %Also sort corresponding (evaluated) vertices 
                       v(:, j) = temp;
                       j = j-1;
                   end
                    %%NM_state = 3;   %Reflection 

                    v_sum = xin*0;  %Initialize sum for mean calculation

                    for i=1:n
                        v_sum = v_sum + v(:, i);
                    end

                    v_m = v_sum*n_r; %Centroid
                    v_r  = v_m*(1+alpha) - alpha*v(:, np1);
                    y  = v_r;
                    NM_state = 4;   %Reflection Evaluate
               else
                   for j=2:n+1   %Shrink
                     v(:,j) = v(:,1)*(1-delta) + delta*v(:,j);
                   end
                   y = v(:, 2);   %Start with evaluation
                   Full_eval_count = 2; 
                   NM_state = 1; %Full vertex evaluation after shrink
               end
            case 7
                f_c = f;%costFunctionJ;
                   if (f_c<fv(np1))
                       v(:, np1) = v_c;
                       fv(np1) = f_c;
                       %NM_state = 2;
                        j = Full_eval_count;  %New value came in, insert it into list
                        while ( (j>1) && (fv(j-1)>fv(j)) ) %Sort ascending
                           temp = fv(j-1);
                           fv(j-1) = fv(j);
                           fv(j) = temp;
                           temp = v(:, j-1);
                           v(:, j-1) = v(:, j); %Also sort corresponding (evaluated) vertices 
                           v(:, j) = temp;
                           j = j-1;
                        end
                        NM_state = 3;   %Reflection 

                        v_sum = xin*0;  %Initialize sum for mean calculation

                        for i=1:n
                            v_sum = v_sum + v(:, i);
                        end

                        v_m = v_sum*n_r; %Centroid
                        v_r  = v_m*(1+alpha) - alpha*v(:, np1);
                        y  = v_r;
    %                     NM_state = 4;   %Reflection Evaluate
                   else
                       for j=2:n+1 %Shrink
                         v(:,j) = v(:,1)*(1-delta) + delta*v(:,j);
                       end
                       y = v(:,2);   %Start with evaluation
                       Full_eval_count = 2; 
                       NM_state = 1; %Full vertex evaluation after shrink  
                   end     
            otherwise
            y = v(:,1);
         end %End switch NM_states   

         %restart window implemented inside the GCNM function

        bufferJ(windowCounter)=v_m(1,1);                                    %centroid window instead cost function (working without noise)
        bufferGamma1(windowCounter)=OV;
        bufferGamma2(windowCounter)=TS;
%         bufferDelta1(windowCounter)=BiasRFState1PowerSetpointError;
%         bufferDelta2(windowCounter)=BiasRFState2PowerSetpointError;
%         bufferPS1(windowCounter)=  ADVCIPulseQualityDeviationState1;
%         bufferPS2(windowCounter)=  ADVCIPulseQualityDeviationState2;

    %      bufferJ(windowCounter)=f; %cost function window 
         windowCounter=windowCounter+1;
         if windowCounter>bufferWindow
            convergenceThresholdStd=(std(bufferJ));
            gamma1Std=(mean(bufferGamma1));
            gamma2Std=(mean(bufferGamma2));
            delta1Std=(mean(bufferDelta1));
            delta2Std=(mean(bufferDelta2));
            ps1Std=(mean(bufferPS1));
            ps2Std=(mean(bufferPS2));

            windowCounter=1;

         end


    else            %this condition appears when the controller is disabled
         y = yp;
         gammaCond=true;
         deltaCond=true;
%          psCond=true;
     
end

%outputs definitions
     yp = y;
     NM_state_val = NM_state;
     centroid= v_m; 
     delay_wait_on_off_z = delay_wait_on_off; 
     %sliding window updating
     convergenceThresholdBuffer=convergenceThresholdStd;      %std
     %buffers constraint condition update
             
        OVBuffer=gamma1Std;
        TSBuffer=gamma2Std;
%         BiasRFState1PowerSetpointErrorBuffer=delta1Std;
%         BiasRFState2PowerSetpointErrorBuffer=delta2Std;
%         ADVCIPulseQualityDeviationState1Buffer=ps1Std;
%         ADVCIPulseQualityDeviationState2Buffer=ps2Std;
%      
     
     
end %End of function

== matlab function ABLF_SOC_benchmark/GCNM/Cost function1/MATLAB Function ==
  settings: updateMethod=DISCRETE
  data: y input; ts output; time input; ovf output; epsilon input; r input; period input
function [ts,ovf] = performance(y,time,epsilon,r,period)
        persistent OV tsFlag
        
          if isempty(OV)        %initialization state
              OV=0;
              tsFlag=1;
%               ts=0;
          end
          
          
          OVCurrent=max(y);
          if OVCurrent>OV
              OV=OVCurrent;
              ovf=OV;
          else
              ovf=OV;
          end
          
          if mod(time,period)==0    %restart constrainst after each repetitive period
            OV=0;
          end
          
          
          if std(y)<epsilon && tsFlag==1 && r==1 %settling time on the low state
              ts=time;
              tsFlag=0;
          else
              ts=5;
          end
          

end
